simulink model "SWC_HALOUT_type"  (R2021b)
settings: Solver=FixedStepDiscrete  StartTime=0.0  StopTime=10.0  FixedStep=0.001  RelTol=1e-3
values from neighbouring files (symbols this model uses):
  DIDLen_APPPedalZP = uint16(3)    [vcu_local_hdr.m]
  DIDLen_APSFunConfig = uint16(16)    [vcu_local_hdr.m]
  DIDLen_AutoLock = uint16(1)    [vcu_local_hdr.m]
  DIDLen_AutoWipHSpdEN = uint16(1)    [vcu_local_hdr.m]
  DIDLen_DKCKey = uint16(8)    [vcu_local_hdr.m]
  DIDLen_DRLDis = uint16(1)    [vcu_local_hdr.m]
  DIDLen_DynoMode = uint16(1)    [vcu_local_hdr.m]
  DIDLen_FMHTimer = uint16(1)    [vcu_local_hdr.m]
  DIDLen_LFLowPresThre = uint16(1)    [vcu_local_hdr.m]
  DIDLen_LFSensorID = uint16(4)    [vcu_local_hdr.m]
  DIDLen_LRLowPresThre = uint16(1)    [vcu_local_hdr.m]
  DIDLen_LRSensorID = uint16(4)    [vcu_local_hdr.m]
  DIDLen_NVMPedalZP = uint16(3)    [vcu_local_hdr.m]
  DIDLen_RFLowPresThre = uint16(1)    [vcu_local_hdr.m]
  DIDLen_RFSensorID = uint16(4)    [vcu_local_hdr.m]
  DIDLen_RRLowPresThre = uint16(1)    [vcu_local_hdr.m]
  DIDLen_RRSensorID = uint16(4)    [vcu_local_hdr.m]
  DIDLen_SensorMode = uint16(1)    [vcu_local_hdr.m]
  DIDLen_TireSize = uint16(16)    [vcu_local_hdr.m]
  DIDLen_TPMSLearnSta = uint16(1)    [vcu_local_hdr.m]
  DIDLen_TurnLampFLThreCurr = uint16(1)    [vcu_local_hdr.m]
  DIDLen_TurnLampFRThreCurr = uint16(1)    [vcu_local_hdr.m]
  DIDLen_TurnLampRLThreCurr = uint16(1)    [vcu_local_hdr.m]
  DIDLen_TurnLampRRThreCurr = uint16(1)    [vcu_local_hdr.m]
  DIDLen_USSConfig = uint16(16)    [vcu_local_hdr.m]
  DIDLen_WhlPres = uint16(4)    [vcu_local_hdr.m]
  DIDLen_WhlSensorBattSta = uint16(1)    [vcu_local_hdr.m]
  DIDLen_WhlTmp = uint16(4)    [vcu_local_hdr.m]
  DIDLen_WipRLSCmdCutFilter = uint16(1)    [vcu_local_hdr.m]
  DIDLen_WipRLSCmdHoldFilter = uint16(1)    [vcu_local_hdr.m]
  DIDLen_XWDMode = uint16(1)    [vcu_local_hdr.m]
  DIDNum_APPPedalZP = uint16(0x0206)    [vcu_local_hdr.m]
  DIDNum_APSFunConfig = uint16(0x0903)    [vcu_local_hdr.m]
  DIDNum_AutoLock = uint16(0x0306)    [vcu_local_hdr.m]
  DIDNum_AutoWipHSpdEN = uint16(0x0308)    [vcu_local_hdr.m]
  DIDNum_DKCKey = uint16(0x0202)    [vcu_local_hdr.m]
  DIDNum_DRLDis = uint16(0x0307)    [vcu_local_hdr.m]
  DIDNum_DynoMode = uint16(0x0203)    [vcu_local_hdr.m]
  DIDNum_FMHTimer = uint16(0x0305)    [vcu_local_hdr.m]
  DIDNum_LFLowPresThre = uint16(0x0B08)    [vcu_local_hdr.m]
  DIDNum_LFSensorID = uint16(0x0B01)    [vcu_local_hdr.m]
  DIDNum_LRLowPresThre = uint16(0x0B0A)    [vcu_local_hdr.m]
  DIDNum_LRSensorID = uint16(0x0B03)    [vcu_local_hdr.m]
  DIDNum_NVMPedalZP = uint16(0x0207)    [vcu_local_hdr.m]
  DIDNum_RFLowPresThre = uint16(0x0B09)    [vcu_local_hdr.m]
  DIDNum_RFSensorID = uint16(0x0B02)    [vcu_local_hdr.m]
  DIDNum_RRLowPresThre = uint16(0x0B0B)    [vcu_local_hdr.m]
  DIDNum_RRSensorID = uint16(0x0B04)    [vcu_local_hdr.m]
  DIDNum_SensorMode = uint16(0x0B0C)    [vcu_local_hdr.m]
  DIDNum_TireSize = uint16(0x0902)    [vcu_local_hdr.m]
  DIDNum_TPMSLearnSta = uint16(0x0B0D)    [vcu_local_hdr.m]
  DIDNum_TurnLampFLThreCurr = uint16(0x0303)    [vcu_local_hdr.m]
  DIDNum_TurnLampFRThreCurr = uint16(0x0301)    [vcu_local_hdr.m]
  DIDNum_TurnLampRLThreCurr = uint16(0x0304)    [vcu_local_hdr.m]
  DIDNum_TurnLampRRThreCurr = uint16(0x0302)    [vcu_local_hdr.m]
  DIDNum_USSConfig = uint16(0x0901)    [vcu_local_hdr.m]
  DIDNum_WhlPres = uint16(0x0B05)    [vcu_local_hdr.m]
  DIDNum_WhlSensorBattSta = uint16(0x0B07)    [vcu_local_hdr.m]
  DIDNum_WhlTmp = uint16(0x0B06)    [vcu_local_hdr.m]
  DIDNum_WipRLSCmdCutFilter = uint16(0x030A)    [vcu_local_hdr.m]
  DIDNum_WipRLSCmdHoldFilter = uint16(0x0309)    [vcu_local_hdr.m]
  DIDNum_XWDMode = uint16(0x0201)    [vcu_local_hdr.m]
  ENUM_TPMSLearnStatus_LEARNED = uint8(  1  )    [vcu_local_hdr.m]
  ENUM_TPMSLearnStatus_LEARNFAIL = uint8(  2  )    [vcu_local_hdr.m]
  ENUM_TPMSLearnStatus_NOTLEARN = uint8(  0  )    [vcu_local_hdr.m]
  FALSE = boolean( 0 )    [vcu_local_hdr.m]    (also in vcu_local_hdrTA2.m)
  TRUE = boolean( 1 )    [vcu_local_hdr.m]    (also in vcu_local_hdrTA2.m)
  ZERO_INT = uint8(0)    [vcu_local_hdr.m]    (also in vcu_local_hdrTA2.m)
undefined symbols (not defined in the file or in its folder): f32_ApsOutVehSpdSig, R_DIDWriteCDD_CSOP_DIDSet_APPPedalZP, R_DIDWriteCDD_CSOP_DIDSet_APSFunConfig, R_DIDWriteCDD_CSOP_DIDSet_AutoLock, R_DIDWriteCDD_CSOP_DIDSet_AutoWipHSpdEN, R_DIDWriteCDD_CSOP_DIDSet_DKCKey, R_DIDWriteCDD_CSOP_DIDSet_DRLDis, R_DIDWriteCDD_CSOP_DIDSet_DynoMode, R_DIDWriteCDD_CSOP_DIDSet_FMHTimer, R_DIDWriteCDD_CSOP_DIDSet_LFLowPresThre, R_DIDWriteCDD_CSOP_DIDSet_LFSensorID, R_DIDWriteCDD_CSOP_DIDSet_LRLowPresThre, R_DIDWriteCDD_CSOP_DIDSet_LRSensorID, R_DIDWriteCDD_CSOP_DIDSet_NVMPedalZP, R_DIDWriteCDD_CSOP_DIDSet_RFLowPresThre, R_DIDWriteCDD_CSOP_DIDSet_RFSensorID, R_DIDWriteCDD_CSOP_DIDSet_RRLowPresThre, R_DIDWriteCDD_CSOP_DIDSet_RRSensorID, R_DIDWriteCDD_CSOP_DIDSet_SensorMode, R_DIDWriteCDD_CSOP_DIDSet_TireSize, R_DIDWriteCDD_CSOP_DIDSet_TPMSLearnSta, R_DIDWriteCDD_CSOP_DIDSet_TurnLampFLThreCurr, R_DIDWriteCDD_CSOP_DIDSet_TurnLampFRThreCurr, R_DIDWriteCDD_CSOP_DIDSet_TurnLampRLThreCurr, R_DIDWriteCDD_CSOP_DIDSet_TurnLampRRThreCurr, R_DIDWriteCDD_CSOP_DIDSet_USSConfig, R_DIDWriteCDD_CSOP_DIDSet_WhlPres, R_DIDWriteCDD_CSOP_DIDSet_WhlSensorBattSta, R_DIDWriteCDD_CSOP_DIDSet_WhlTmp, R_DIDWriteCDD_CSOP_DIDSet_WipRLSCmdCutFilter, R_DIDWriteCDD_CSOP_DIDSet_WipRLSCmdHoldFilter, R_DIDWriteCDD_CSOP_DIDSet_XWDMode, R_FDCCDD_Inner_CSOP_FDC_AppCallSleep, R_HALINCDD_CSOP_PAS_Handler, R_HALINCDD_CSOP_UDS_Main, R_HALOUT_APS_CSOP_ApsOutput, R_HALOUTCDD_CSOP_AppNmStateReq, R_HALOUTCDD_CSOP_ResetPedalZeroPosDone, R_HALOUTCDD_CSOP_SetAcoreRebootCmdACK, R_HALOUTCDD_CSOP_SetHazardIND, R_HALOUTCDD_CSOP_SetSysPwrStat, R_HALOUTCDD_CSOP_SleepRequest, R_HALOUTCDD_CSOP_TPMSSensorIDRegSetResults, R_IOExpOUT_CDD_CSOP_IOExpSetVal, R_J1939_CAN1_FD1_CE100_0_CSOP_Write_CAN1_FD1_CE100_0, R_J1939_CAN1_FD1_CE100_1_CSOP_Write_CAN1_FD1_CE100_1, R_NVMWriteCDD_Inner_NVM_WriteOperation, R_UDSCDD_CSOP_DdmRestartOperationCycle, R_WDGCDD_CSOP_Call_WDG_AppEnd, u16_DIDLen_APPPedalZP, u16_DIDLen_APSFunConfig, u16_DIDLen_AutoLock, u16_DIDLen_AutoWipHSpdEN, u16_DIDLen_DKCKey, u16_DIDLen_DRLDis, u16_DIDLen_DynoMode, u16_DIDLen_FMHTimer, u16_DIDLen_LFLowPresThre, u16_DIDLen_LFSensorID, u16_DIDLen_LRLowPresThre ... (+95)
libraries: FVT_lib x142, simulink x107, hdlsllib x6, hcu_lib x5, halout x1
(part 2 of 8)

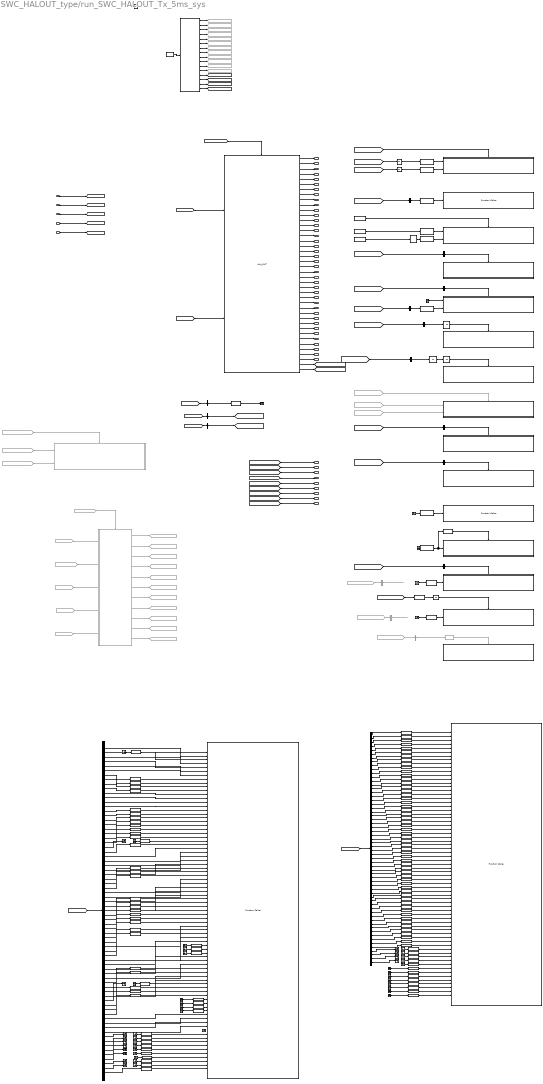
== system SWC_HALOUT_type/run_SWC_HALOUT_Tx_5ms_sys ==
  R_BSCP_outputs_BSCP_outputs_read : Inport
  R_BOUTP_outputs_BOUTP_outputs_read : Inport  Port=2
  R_BHAL_SYS_outputs_BHAL_SYS_outputs_read : Inport  Port=3
  R_BHAL_DID_outputs_BHAL_DID_outputs_read : Inport  Port=4
  R_NVMReadCDD_u8Array1024_NVMReadData_read : Inport  Port=5
  function : TriggerPort  TriggerType=function-call  VariantControl=(inherit)  SampleTimeType=periodic  SampleTime=-1
  Bus Selector1 : BusSelector  OutputSignals=VOUTP_triggerBAM_flg
  Bus Selector15 : BusSelector  OutputSignals=VHAL_AcoreReadyToSlp_flg
  Bus Selector2 : BusSelector  OutputSignals=VOUTP_triggerDT_flg
  Bus Selector3 : BusSelector  OutputSignals=VOUTP_BrkPedalPos_pct,VOUTP_ActAPSPosn_pct,VOUTP_LFRawWhlSpeed_kph,VOUTP_RFRawWhlSpeed_kph,VOUTP_LRRawWhlSpeed_kph,VOUTP_RRRawWhlSpeed_kph,VOUTP_LFRawWhlSpeedV_flg,VOUTP_RFRawWhlSpeedV_flg,VOUTP_LRRawWhlSpeedV_flg,VOUTP_RRRawWhlSpeedV_flg,VOUTP_LFWhlRotDir_enum,VOUTP_RFWhlRotDir_enum,VOUTP_LRWhlRotDir_enum,VOUTP_RRWhlRotDir_enum,VOUTP_LFPulseCountV_flg,VOUTP_RFPulseCountV_flg,VOUTP_LRPulseCountV_flg,VOUTP_RRPulseCountV_flg,VOUTP_LFPulseCount_enum,VOUTP_RFPulseCount_enum,VOUTP_LRPulseCount_enum,VOUTP_RRPulseCount_enum,VOUTP_VehSpeed_kph,VOUTP_APSCtrlAvail_flg,VOUTP_ShifterHandleCmd_enum,VOUTP_DriIntend_enum,VOUTP_EPSAOIControl_enum,VOUTP_SASAngle_Deg,VOUTP_SASSpeed_degps,VOUTP_SASSpeedValid_flg,VOUTP_SASCAL_flg,VOUTP_SASV_flg,VOUTP_GRADE_Deg,VOUTP_YawRate_degps,VOUTP_LatAccel_Gps,VOUTP_LongAccel_Gps,VOUTP_MCPressure_bar,VOUTP_YawRateV_flg,VOUTP_LatAccelV_flg,VOUTP_LongAccelV_flg,VOUTP_MCPressureV_bar,VOUTP_BrkSwSta_flg,VOUTP_BrkSwV_flg,VOUTP_ESCStandstill_flg,VOUTP_ESCAPSSta_enum,VOUTP_EPBExtReleaseAvail_flg,VOUTP_EPBExtApplyAvail_flg,VOUTP_EPBErrSta_enum,VOUTP_EPBSta_enum,VOUTP_AVMparkingcancel_enum,VOUTP_AVMparkingexcute_enum,VOUTP_AVMParkingmode_enum,VOUTP_AVMErrSTA_flg,VOUTP_IVIStatus_flg,VOUTP_CAASSw_enum,VOUTP_IVIScreen_enum,VOUTP_VehSpeedTimeOut_flg,VOUTP_ABSActive_flg,VOUTP_TCSActive_flg,VOUTP_DriverSeatBeltCmd_flg,VOUTP_RFPressIndi_enum,VOUTP_LFPressIndi_enum,VOUTP_RRPressIndi_enum,VOUTP_LRPressIndi_enum,VOUTP_FSOffSw_enum,VOUTP_FSOffSwTimeOut_flg,VOUTP_VehSpeed_kph,VOUTP_VehSpeed_kph,VOUTP_VehSpeed_kph,VOUTP_VehSpeed_kph,VOUTP_VehSpeed_kph,VOUTP_VehSpeed_kph,VOUTP_IVIUserTakeOverAPSSta_flg
  Bus Selector4 : BusSelector  OutputSignals=VOUTP_BrkPedalPosTimeOut_flg,VOUTP_LFRawWhlSpeedTimeOut_flg,VOUTP_RFRawWhlSpeedTimeOut_flg,VOUTP_LRRawWhlSpeedTimeOut_flg,VOUTP_RRRawWhlSpeedTimeOut_flg,VOUTP_LFRawWhlSpeedVTimeOut_flg,VOUTP_RFRawWhlSpeedVTimeOut_flg,VOUTP_LRRawWhlSpeedVTimeOut_flg,VOUTP_RRRawWhlSpeedVTimeOut_flg,VOUTP_LFWhlRotDirTimeOut_flg,VOUTP_RFWhlRotDirTimeOut_flg,VOUTP_LRWhlRotDirTimeOut_flg,VOUTP_RRWhlRotDirTimeOut_flg,VOUTP_LFPulseCountVTimeOut_flg,VOUTP_RFPulseCountVTimeOut_flg,VOUTP_LRPulseCountVTimeOut_flg,VOUTP_RRPulseCountVTimeOut_flg,VOUTP_LFPulseCountTimeOut_flg,VOUTP_RFPulseCountTimeOut_flg,VOUTP_LRPulseCountTimeOut_flg,VOUTP_RRPulseCountTimeOut_flg,VOUTP_ShifterHandleCmdTimeOut_flg,VOUTP_DriIntendTimeOut_flg,VOUTP_EPSAOIControlTimeOut_flg,VOUTP_SASAngleTimeOut_flg,VOUTP_SASSpeedTimeOut_flg,VOUTP_SASSpeedValidTimeOut_flg,VOUTP_SASCALTimeOut_flg,VOUTP_SASVTimeOut_flg,VOUTP_GRADETimeOut_flg,VOUTP_YawRateTimeOut_flg,VOUTP_LatAccelTimeOut_flg,VOUTP_LongAccelTimeOut_flg,VOUTP_MCPressureTimeOut_flg,VOUTP_YawRateVTimeOut_flg,VOUTP_LatAccelVTimeOut_flg,VOUTP_LongAccelVTimeOut_flg,VOUTP_MCPressureVTimeOut_flg,VOUTP_BrkSwStaTimeOut_flg,VOUTP_BrkSwVTimeOut_flg,VOUTP_ESCStandstillTimeOut_flg,VOUTP_ESCAPSStaTimeOut_flg,VOUTP_EPBExtReleaseAvailTimeOut_flg,VOUTP_EPBExtApplyAvailTimeOut_flg,VOUTP_EPBErrStaTimeOut_flg,VOUTP_EPBStaTimeOut_flg,VOUTP_AVMparkingcancelTimeOut_flg,VOUTP_AVMparkingexcuteTimeOut_flg,VOUTP_AVMParkingmodeTimeOut_flg,VOUTP_AVMErrSTATimeOut_flg,VOUTP_IVIStatusTimeOut_flg,VOUTP_CAASSwTimeOut_flg,VOUTP_IVIScreenTimeOut_flg,VOUTP_ABSActiveTimeOut_flg,VOUTP_TCSActiveTimeOut_flg,VOUTP_DriverSeatBeltCmdTimeOut_flg,VOUTP_RFPressIndi_enum,VOUTP_LFPressIndi_enum,VOUTP_RRPressIndi_enum,VOUTP_LRPressIndi_enum
  Bus Selector6 : BusSelector  Commented=on  OutputSignals=VHAL_TPMSSensorIDRegResults_raw8
  Bus Selector8 : BusSelector  Commented=on  OutputSignals=VOUTP_ResetPedalZeroPosStart_flg
  Bus Selector9 : BusSelector  Commented=on  OutputSignals=VHAL_DIDSetNVMPedalZP_raw8
  Constant2 : Constant  Value=TRUE
  Constant3 : Constant  Value=TRUE
  Constant4 : Constant  Value=TRUE
  Constant5 : Constant  Value=FALSE
  DIDSet_Subsystem : Subsystem  Commented=on
  DIDSet_Subsystem1 : From  Commented=on  GotoTag=BOUTP_DIDSetData_outputs
  DIDSet_Subsystem2 : From  Commented=on  GotoTag=BHAL_DID_outputs
  DIDSet_Subsystem3 : From  Commented=on  GotoTag=trig_SetDID
  Data Type Conversion{,1..2,4..5,7..13,17..19,21..107,109..125,128..130} (122 alike) : DataTypeConversion  OutDataTypeStr=uint8
  Data Type Conversion108 : DataTypeConversion  OutDataTypeStr=boolean
  Data Type Conversion126 : DataTypeConversion  OutDataTypeStr=boolean
  Data Type Conversion127 : DataTypeConversion  OutDataTypeStr=boolean
  Data Type Conversion{14..16,20} (4 alike) : DataTypeConversion  OutDataTypeStr=int16
  Data Type Conversion3 : DataTypeConversion  OutDataTypeStr=uint32
  Data Type Conversion6 : DataTypeConversion  OutDataTypeStr=single
  Detect Increase1 : simulink/Logic and Bit Operations/Detect Increase  Commented=on  vinit=0.0  OutDataTypeStr=boolean
  From104 : From  Commented=on  GotoTag=BHAL_SYS_outputs
  From118 : From  Commented=on  GotoTag=BHAL_SYS_outputs
  From121 : From  Commented=on  GotoTag=trig_OUTP_AFTER_40_1
  From122 : From  Commented=on  GotoTag=BOUTP_outputs
  From134 : From  Commented=on  GotoTag=BOUTP_DIDSetData_outputs
  From139 : From  Commented=on  GotoTag=BOUTP_outputs
  From144 : From  Commented=on  GotoTag=BOUTP_DIDSetData_outputs
  From18 : From  Commented=on  GotoTag=Header_Array
  From19 : From  Commented=on  GotoTag=DTC_Array
  From20 : From  Commented=on  GotoTag=DTC_Trigger
  From35 : From  Commented=on  GotoTag=u8Array1024_NvmReadArray
  From36 : From  Commented=on  GotoTag=BHAL_DID_outputs
  Goto10 : Goto  Commented=on  GotoTag=u8Array1024_NvmWriteArray
  Goto100 : Goto  Commented=on  GotoTag=trig_Read_NVM_00
  Goto102 : Goto  Commented=on  GotoTag=trig_ReadIMUOffset_00
  Goto105 : Goto  Commented=on  GotoTag=u8_ApsOutSetFrSensorOnCmd
  Goto106 : Goto  Commented=on  GotoTag=trig_GetNMID
  Goto107 : Goto  Commented=on  GotoTag=u8_ApsOutSetFrSensorSwTOCmd
  Goto108 : Goto  Commented=on  GotoTag=u8_ApsOutSetVehSpdTOCmd
  Goto109 : Goto  Commented=on  GotoTag=Header_Array
  Goto110 : Goto  Commented=on  GotoTag=u8_ApsOutSendChrgPlugSta
  Goto111 : Goto  Commented=on  GotoTag=f32_ApsOutVehSpdSig
  Goto113 : Goto  Commented=on  GotoTag=DTC_Array
  Goto119 : Goto  Commented=on  GotoTag=trig_HAL_DKC_10_3
  Goto121 : Goto  Commented=on  GotoTag=DTC_Trigger
  Goto122 : Goto  Commented=on  GotoTag=u8_ApsOutGearPosnSig
  Goto124 : Goto  Commented=on  GotoTag=BOUTP_DIDSetData_outputs
  Goto90 : Goto  Commented=on  GotoTag=trig_GetDID
  Goto91 : Goto  Commented=on  GotoTag=trig_WDG
  Goto92 : Goto  Commented=on  GotoTag=trig_HAL_DKC_10_2
  Goto93 : Goto  Commented=on  GotoTag=trig_HAL_CDD_10_1
  Goto96 : Goto  Commented=on  GotoTag=trig_OUTP_40
  Goto97 : Goto  Commented=on  GotoTag=trig_APP_30
  Goto98 : Goto  Commented=on  GotoTag=trig_INP_20
  Goto99 : Goto  Commented=on  GotoTag=trig_HAL_IN_10
  Ground{,1..18,20..21} (21 alike) : Ground
  Ground_{1,11..14,16..24,26,36..37} (17 alike) : Ground
  HALOUT_AFTER : Subsystem
  HAL_OUT : halout/HAL_OUT  SystemSampleTime=-1  VariantActivationTime=update diagram  Latency=0  AutoFrameSizeCalculation=off
  NOT : Logic  Operator=NOT  Inputs=1  AllPortsSameDT=off  OutDataTypeStr=boolean
  OUTP_AFTER : Subsystem  Commented=on
      settings: RTWSystemCode=Nonreusable function  RTWFcnNameOpts=Use subsystem name  RTWFileNameOpts=Use subsystem name
  R_DIDWriteCDD_CSOP_DIDSet_NVMPedalZP : Subsystem
  R_FDCCDD_Inner_CSOP_FDC_AppCallSleep : Subsystem
  R_HALOUTCDD_CSOP_AppNmStateReq : Subsystem
  R_HALOUTCDD_CSOP_ResetPedalZeroPosDone : Subsystem
  R_HALOUTCDD_CSOP_SetAcoreRebootCmdACK : Subsystem
  R_HALOUTCDD_CSOP_SetHazardIND : FunctionCaller  FunctionPrototype=R_HALOUTCDD_CSOP_SetHazardIND(u8_HazardIND)  InputArgumentSpecifications=uint8(1)
  R_HALOUTCDD_CSOP_SetSysPwrStat : FunctionCaller  FunctionPrototype=R_HALOUTCDD_CSOP_SetSysPwrStat(u8_SysPwrStat)  InputArgumentSpecifications=uint8(1)
  R_HALOUTCDD_CSOP_SleepRequest : Subsystem
  R_HALOUTCDD_CSOP_TPMSSensorIDRegSetResults : Subsystem
  R_HALOUT_APS_CSOP_ApsSetData : FunctionCaller  FunctionPrototype=R_HALOUT_APS_CSOP_ApsSetData(u8_SetPwrSta,f32_SetBrkPedalPos,f32_SetActAPSPosn,f32_SetLF_RawWhlSpeed,f32_SetRF_RawWhlSpeed,f32_SetLR_RawWhlSpeed,f32_SetRR_RawWhlSpeed,u8_SetLF_RawWhlSpeed_V,u8_SetRF_RawWhlSpeed_V,u8_SetLR_RawWhlSpeed_V,u8_SetRR_RawWhlSpeed_V,u8_SetLF_WhlRotDir,u8_SetRF_WhlRotDir,u8_SetLR_WhlRotDir,u8_SetRR_WhlRotDir,u8_SetLF_PulseCount_V,u8_SetRF_PulseCount_V,u8_SetLR_PulseCount_V,u8_SetRR_PulseCount_V,s16_SetLF_PulseCount,s16_SetRF_PulseCount,s16_SetLR_PulseCount,s16_SetRR_PulseCount,u8_SetAPS_Active,u8_SetAPS_CtrlAvail,u8_SetShifter_Handle_Cmd,u8_SetDriIntend,u8_SetEPS_AOI_Control,f32_SetSAS_Angle,f32_SetSAS_Speed,u8_SetSAS_Speed_Valid,u8_SetSAS_CAL,u8_SetSAS_OK,f32_SetGRADE,f32_SetYawRate,f32_SetLatAccel,f32_SetLongAccel,f32_SetMCPressure,u8_SetYawRate_V,u8_SetLatAccel_V,u8_SetLongAccel_V,u8_SetMCPressure_V,u8_SetBrkSw_Sta,u8_SetBrkSw_V,u8_SetESC_Standstill,u8_SetESC_APS_Sta,u8_SetEPBExtReleaseAvail,u8_SetEPBExtApplyAvail,u8_SetEPBErrSta,u8_SetEPBSta,u8_SetAllDoorSW,u8_SetHoodSW,u8_SetTailgate_SW,u8_SetAVM_parking_cancel,u8_SetAVM_parking_excute,u8_SetAVM_Parking_mode,u8_SetAVM_Err_STA,u8_SetIVI_Status,u8_SetCAAS_Sw,u8_SetIVI_Screen,u8_SetCAAS_CtrlAvail,u8_SetABS_Active,u8_SetTCS_Active,u8_SetDriverSeatBeltCmd,u8_SetDrDoorSW,u8_SetPsDoorSW,u8_SetRLDoorSW,u8_SetRRDoorSW,u8_SetRFPressIndi,u8_SetLFPressIndi,u8_SetRRPressIndi,u8_SetLRPressIndi,f32_SetsigAmbAirT,f32_SetVehActSpd,u8_SetCAAS_Active,u8_SetAPS_PwrReqAvail_sta,u8_SetDKC_PDkeyAreaRAPS_Sta,u8_SetDKC_ParkingMode_Cmd,u8_SetP_UID_LowPower,u8_SetDr_SeatSta,u8_SetVCU_RAPSErrLv2_flg,u8_SetVCU_RAPSErrLv3_flg,u8_SetIVI_UserTakeOver_APS_Sta)  InputArgumentSpecifications=uint8(1), single(1), single(1), single(1), single(1), single(1), single(1), uint8(1), uint8(1), uint8(1), uint8(1), uint8(1), uint8(1), uint8(1), uint8(1), uint8(1), uint8(1), uint8(1), uint8(1), int16(1), int16(1), int16(1), int16(1), uint8(1), uint8(1), uint8(1), uint8(1), uint8(1), single(1), single(1), uint8(1), uint8(1), uint8(1), single(1), single(1), single(1), single(1), single(1), uint8(1), uint8(1), uint8(1), uint8(1), uint8(1), uint8(1), uint8(1), uint8(1), uint8(1), uint8(1), uint8(1), uint8(1), uint8(1), uint8(1), uint8(1), uint8(1), uint8(1), uint8(1), uint8(1), uint8(1), uint8(1), uint8(1), uint8(1), uint8(1), uint8(1), uint8(1), uint8(1), uint8(1), uint8(1), uint8(1), uint8(1), uint8(1), uint8(1), uint8(1), single(1), single(1), uint8(1), uint8(1), uint8(1), uint8(1), uint8(1), uint8(1), uint8(1), uint8(1), uint8(1)
  R_HALOUT_APS_CSOP_ApsSetTimeout : FunctionCaller  FunctionPrototype=R_HALOUT_APS_CSOP_ApsSetTimeout(u8_SetBrkPedalPosTO,u8_SetLF_RawWhlSpeedTO,u8_SetRF_RawWhlSpeedTO,u8_SetLR_RawWhlSpeedTO,u8_SetRR_RawWhlSpeedTO,u8_SetLF_RawWhlSpeed_VTO,u8_SetRF_RawWhlSpeed_VTO,u8_SetLR_RawWhlSpeed_VTO,u8_SetRR_RawWhlSpeed_VTO,u8_SetLF_WhlRotDirTO,u8_SetRF_WhlRotDirTO,u8_SetLR_WhlRotDirTO,u8_SetRR_WhlRotDirTO,u8_SetLF_PulseCount_VTO,u8_SetRF_PulseCount_VTO,u8_SetLR_PulseCount_VTO,u8_SetRR_PulseCount_VTO,u8_SetLF_PulseCountTO,u8_SetRF_PulseCountTO,u8_SetLR_PulseCountTO,u8_SetRR_PulseCountTO,u8_SetShifter_Handle_CmdTO,u8_SetDriIntendTO,u8_SetEPS_AOI_ControlTO,u8_SetSAS_AngleTO,u8_SetSAS_SpeedTO,u8_SetSAS_Speed_ValidTO,u8_SetSAS_CALTO,u8_SetSAS_OKTO,u8_SetGRADETO,u8_SetYawRateTO,u8_SetLatAccelTO,u8_SetLongAccelTO,u8_SetMCPressureTO,u8_SetYawRate_VTO,u8_SetLatAccel_VTO,u8_SetLongAccel_VTO,u8_SetMCPressure_VTO,u8_SetBrkSw_StaTO,u8_SetBrkSw_VTO,u8_SetESC_StandstillTO,u8_SetESC_APS_StaTO,u8_SetEPBExtReleaseAvailTO,u8_SetEPBExtApplyAvailTO,u8_SetEPBErrStaTO,u8_SetEPBStaTO,u8_SetAVM_parking_cancelTO,u8_SetAVM_parking_excuteTO,u8_SetAVM_Parking_modeTO,u8_SetAVM_Err_STATO,u8_SetIVI_StatusTO,u8_SetCAAS_SwTO,u8_SetIVI_ScreenTO,u8_SetABS_ActiveTO,u8_SetTCS_ActiveTO,u8_SetDriverSeatBeltCmdTO,u8_SetRFPressIndiTO,u8_SetLFPressIndiTO,u8_SetRRPressIndiTO,u8_SetLRPressIndiTO,u8_SetsigAmbAirTTO,u8_SetAPS_PwrReqAvail_staTO,u8_SetDKC_PDkeyAreaRAPS_StaTO,u8_SetDKC_ParkingMode_CmdTO,u8_SetP_UID_LowPowerTO,u8_SetDr_SeatStaTO,u8_SetVCU_RAPSErrLv2_flgTO,u8_SetVCU_RAPSErrLv3_flgTO,u8_SetIVI_UserTakeOver_APS_StaTO)  InputArgumentSpecifications=uint8(1), uint8(1), uint8(1), uint8(1), uint8(1), uint8(1), uint8(1), uint8(1), uint8(1), uint8(1), uint8(1), uint8(1), uint8(1), uint8(1), uint8(1), uint8(1), uint8(1), uint8(1), uint8(1), uint8(1), uint8(1), uint8(1), uint8(1), uint8(1), uint8(1), uint8(1), uint8(1), uint8(1), uint8(1), uint8(1), uint8(1), uint8(1), uint8(1), uint8(1), uint8(1), uint8(1), uint8(1), uint8(1), uint8(1), uint8(1), uint8(1), uint8(1), uint8(1), uint8(1), uint8(1), uint8(1), uint8(1), uint8(1), uint8(1), uint8(1), uint8(1), uint8(1), uint8(1), uint8(1), uint8(1), uint8(1), uint8(1), uint8(1), uint8(1), uint8(1), uint8(1), uint8(1), uint8(1), uint8(1), uint8(1), uint8(1), uint8(1), uint8(1), uint8(1)
  R_IOExpOUT_CDD_CSOP_IOExpSetVal : Subsystem
  R_NVMWriteCDD_Inner_NVM_WriteOperation : Subsystem
  R_UDSCDD_CSOP_DdmRestartOperationCycle : Subsystem
  R_UDSCDD_CSOP_SetDTCStatus : Subsystem
  R_WDGCDD_CSOP_Call_WDG_AppEnd : Subsystem
  Terminator{,1..8,10..15} (15 alike) : Terminator
  Unit Delay{,1..5} (6 alike) : UnitDelay  SampleTime=-1  HasFrameUpgradeWarning=on
  bus_selector : BusSelector  OutputSignals=VOUTP_SysPowerMode_enum
  bus_selector10 : BusSelector  OutputSignals=VOUTP_AcoreRebootCmdACK_flg
  bus_selector14 : BusSelector  OutputSignals=VOUTP_TPMSSensorIDRegStart_flg
  bus_selector4 : BusSelector  OutputSignals=VOUTP_NvWriteReqRisingEdge_flg
  bus_selector5 : BusSelector  OutputSignals=VOUTP_FdcSlpTime_sec
  bus_selector6 : BusSelector  OutputSignals=VOUTP_FdcSlpReqRisingEdge_flg
  bus_selector7 : BusSelector  OutputSignals=VOUTP_FdcSlpReqRisingEdge_flg
  bus_selector8 : BusSelector  OutputSignals=VOUTP_FdcSlpReqRisingEdge_flg
  bus_selector9 : BusSelector  OutputSignals=VOUTP_EnterNewOperCyc_flg
  detect_change1 : simulink/Logic and Bit Operations/Detect Change  vinit=0  OutDataTypeStr=boolean
  hcu_main_sched : Stateflow chart  TreatAsAtomicUnit=on
  P_CAN1_FD1_CE100_2_CAN1_SG_FD1_CE100_2_write : Outport
  P_CAN2_FD2_CE100_0_CAN2_SG_FD2_CE100_0_write : Outport  Port=2
  P_CAN4_FD4_CE100_0_CAN4_SG_FD4_CE100_0_write : Outport  Port=3
  P_CAN4_FD4_CE100_1_CAN4_SG_FD4_CE100_1_write : Outport  Port=4
  P_CAN7_FD7_CE100_0_CAN7_SG_FD7_CE100_0_write : Outport  Port=5
  IRV_ms10_CAN1_SG_FD1_C10_0_write : Outport  Port=6  OutDataTypeStr=Bus: DT_CAN1_SG_FD1_C10_0  PortDimensions=1  BusOutputAsStruct=on
  IRV_ms10_CAN1_SG_FD1_C10_1_write : Outport  Port=7  OutDataTypeStr=Bus: DT_CAN1_SG_FD1_C10_1  PortDimensions=1  BusOutputAsStruct=on
  IRV_ms10_CAN2_SG_FD2_C10_0_write : Outport  Port=8  OutDataTypeStr=Bus: DT_CAN2_SG_FD2_C10_0  PortDimensions=1  BusOutputAsStruct=on
  IRV_ms10_CAN3_SG_FD3_C10_0_write : Outport  Port=9  OutDataTypeStr=Bus: DT_CAN3_SG_FD3_C10_0  PortDimensions=1  BusOutputAsStruct=on
  IRV_ms10_CAN3_SG_FD3_C10_1_write : Outport  Port=10  OutDataTypeStr=Bus: DT_CAN3_SG_FD3_C10_1  PortDimensions=1  BusOutputAsStruct=on
  IRV_ms10_CAN4_SG_FD4_C10_0_write : Outport  Port=11  OutDataTypeStr=Bus: DT_CAN4_SG_FD4_C10_0  PortDimensions=1  BusOutputAsStruct=on
  IRV_ms10_CAN7_SG_FD7_C10_0_write : Outport  Port=12  OutDataTypeStr=Bus: DT_CAN7_SG_FD7_C10_0  PortDimensions=1  BusOutputAsStruct=on
  IRV_ms100_CAN1_SG_FD1_C100_0_write : Outport  Port=13  OutDataTypeStr=Bus: DT_CAN1_SG_FD1_C100_0  PortDimensions=1  BusOutputAsStruct=on
  IRV_ms100_CAN1_SG_FD1_C100_1_write : Outport  Port=14  OutDataTypeStr=Bus: DT_CAN1_SG_FD1_C100_1  PortDimensions=1  BusOutputAsStruct=on
  IRV_ms100_CAN1_SG_FD1_C100_2_write : Outport  Port=15  OutDataTypeStr=Bus: DT_CAN1_SG_FD1_C100_2  PortDimensions=1  BusOutputAsStruct=on
  IRV_ms100_CAN1_SG_FD1_C100_3_write : Outport  Port=16  OutDataTypeStr=Bus: DT_CAN1_SG_FD1_C100_3  PortDimensions=1  BusOutputAsStruct=on
  IRV_ms100_CAN2_SG_GW2_C100_0_write : Outport  Port=17  OutDataTypeStr=Bus: DT_CAN2_SG_GW2_C100_0  PortDimensions=1  BusOutputAsStruct=on
  IRV_ms100_CAN3_SG_FD3_C100_0_write : Outport  Port=18  OutDataTypeStr=Bus: DT_CAN3_SG_FD3_C100_0  PortDimensions=1  BusOutputAsStruct=on
  IRV_ms100_CAN4_SG_FD4_C100_0_write : Outport  Port=19  OutDataTypeStr=Bus: DT_CAN4_SG_FD4_C100_0  PortDimensions=1  BusOutputAsStruct=on
  IRV_ms100_CAN5_SG_FD5_C100_0_write : Outport  Port=20  OutDataTypeStr=Bus: DT_CAN5_SG_FD5_C100_0  PortDimensions=1  BusOutputAsStruct=on
  IRV_ms100_CAN7_SG_FD7_C100_0_write : Outport  Port=21  OutDataTypeStr=Bus: DT_CAN7_SG_FD7_C100_0  PortDimensions=1  BusOutputAsStruct=on
  IRV_ms1000_CAN2_SG_FD2_C1000_0_write : Outport  Port=22  OutDataTypeStr=Bus: DT_CAN2_SG_FD2_C1000_0  PortDimensions=1  BusOutputAsStruct=on
  IRV_ms20_CAN1_SG_FD1_C20_0_write : Outport  Port=23  OutDataTypeStr=Bus: DT_CAN1_SG_FD1_C20_0  PortDimensions=1  BusOutputAsStruct=on
  IRV_ms200_CAN1_SG_FD1_C200_0_write : Outport  Port=24  OutDataTypeStr=Bus: DT_CAN1_SG_FD1_C200_0  PortDimensions=1  BusOutputAsStruct=on
  IRV_ms200_CAN2_SG_FD2_C200_0_write : Outport  Port=25  OutDataTypeStr=Bus: DT_CAN2_SG_FD2_C200_0  PortDimensions=1  BusOutputAsStruct=on
  IRV_ms200_CAN3_SG_FD3_C200_0_write : Outport  Port=26  OutDataTypeStr=Bus: DT_CAN3_SG_FD3_C200_0  PortDimensions=1  BusOutputAsStruct=on
  IRV_ms200_CAN3_SG_FD3_C200_1_write : Outport  Port=27  OutDataTypeStr=Bus: DT_CAN3_SG_FD3_C200_1  PortDimensions=1  BusOutputAsStruct=on
  IRV_ms200_CAN4_SG_FD4_C200_0_write : Outport  Port=28  OutDataTypeStr=Bus: DT_CAN4_SG_FD4_C200_0  PortDimensions=1  BusOutputAsStruct=on
  IRV_ms200_CAN5_SG_FD5_C200_0_write : Outport  Port=29  OutDataTypeStr=Bus: DT_CAN5_SG_FD5_C200_0  PortDimensions=1  BusOutputAsStruct=on
  IRV_ms200_CAN6_SG_FD6_C200_0_write : Outport  Port=30  OutDataTypeStr=Bus: DT_CAN6_SG_FD6_C200_0  PortDimensions=1  BusOutputAsStruct=on
  IRV_ms200_CAN7_SG_FD7_C200_0_write : Outport  Port=31  OutDataTypeStr=Bus: DT_CAN7_SG_FD7_C200_0  PortDimensions=1  BusOutputAsStruct=on
  IRV_ms250_CAN1_SG_FD1_C250_0_write : Outport  Port=32  OutDataTypeStr=Bus: DT_CAN1_SG_FD1_C250_0  PortDimensions=1  BusOutputAsStruct=on
  IRV_ms50_CAN1_SG_FD1_C50_0_write : Outport  Port=33  OutDataTypeStr=Bus: DT_CAN1_SG_FD1_C50_0  PortDimensions=1  BusOutputAsStruct=on
  IRV_ms50_CAN1_SG_FD1_C50_1_write : Outport  Port=34  OutDataTypeStr=Bus: DT_CAN1_SG_FD1_C50_1  PortDimensions=1  BusOutputAsStruct=on
  IRV_ms50_CAN2_SG_FD2_C50_0_write : Outport  Port=35  OutDataTypeStr=Bus: DT_CAN2_SG_FD2_C50_0  PortDimensions=1  BusOutputAsStruct=on
  IRV_ms50_CAN7_SG_FD7_C50_0_write : Outport  Port=36  OutDataTypeStr=Bus: DT_CAN7_SG_FD7_C50_0  PortDimensions=1  BusOutputAsStruct=on
  IRV_ms500_CAN2_SG_FD2_C500_0_write : Outport  Port=37  OutDataTypeStr=Bus: DT_CAN2_SG_FD2_C500_0  PortDimensions=1  BusOutputAsStruct=on
  IRV_ms5000_CAN1_SG_FD1_C5000_0_write : Outport  Port=38  OutDataTypeStr=Bus: DT_CAN1_SG_FD1_C5000_0  PortDimensions=1  BusOutputAsStruct=on
  IRV_ms5000_CAN1_SG_FD1_C5000_1_write : Outport  Port=39  OutDataTypeStr=Bus: DT_CAN1_SG_FD1_C5000_1  PortDimensions=1  BusOutputAsStruct=on
  IRV_ms80_CAN1_SG_FD1_C80_0_write : Outport  Port=40  OutDataTypeStr=Bus: DT_CAN1_SG_FD1_C80_0  PortDimensions=1  BusOutputAsStruct=on
  IRV_f32_ApsOutVehSpdSig_write : Outport  Port=41  OutDataTypeStr=single  PortDimensions=1
  IRV_u8Array1024_NvmWriteArray_write : Outport  Port=42  OutDataTypeStr=uint8  PortDimensions=1024
  IRV_u8_ApsOutGearPosnSig_write : Outport  Port=43  OutDataTypeStr=uint8  PortDimensions=1
  IRV_u8_ApsOutSendChrgPlugSta_write : Outport  Port=44  OutDataTypeStr=uint8  PortDimensions=1
  IRV_u8_ApsOutSetFrSensorOnCmd_write : Outport  Port=45  OutDataTypeStr=uint8  PortDimensions=1
  IRV_u8_ApsOutSetFrSensorSwTOCmd_write : Outport  Port=46  OutDataTypeStr=uint8  PortDimensions=1
  IRV_u8_ApsOutSetVehSpdTOCmd_write : Outport  Port=47  OutDataTypeStr=uint8  PortDimensions=1
  IRV_J1939_CAN1_SG_FD1_CE100_0_write : Outport  Port=48  OutDataTypeStr=Bus: DT_CAN1_SG_FD1_CE100_0  PortDimensions=1  BusOutputAsStruct=on
  IRV_J1939_CAN1_SG_FD1_CE100_1_write : Outport  Port=49  OutDataTypeStr=Bus: DT_CAN1_SG_FD1_CE100_1  PortDimensions=1  BusOutputAsStruct=on
  wires:
  [f32_ApsOutVehSpdSig] -> IRV_f32_ApsOutVehSpdSig_write/1
  [u8Array1024_NvmWriteArray] -> IRV_u8Array1024_NvmWriteArray_write/1
  [u8_ApsOutGearPosnSig] -> IRV_u8_ApsOutGearPosnSig_write/1
  [u8_ApsOutSendChrgPlugSta] -> IRV_u8_ApsOutSendChrgPlugSta_write/1
  [u8_ApsOutSetFrSensorOnCmd] -> IRV_u8_ApsOutSetFrSensorOnCmd_write/1
  [u8_ApsOutSetFrSensorSwTOCmd] -> IRV_u8_ApsOutSetFrSensorSwTOCmd_write/1
  [u8_ApsOutSetVehSpdTOCmd] -> IRV_u8_ApsOutSetVehSpdTOCmd_write/1
  [J1939_CAN1_SG_FD1_CE100_0] -> IRV_J1939_CAN1_SG_FD1_CE100_0_write/1
  [J1939_CAN1_SG_FD1_CE100_1] -> IRV_J1939_CAN1_SG_FD1_CE100_1_write/1
  Data Type Conversion/1 -> R_HALOUTCDD_CSOP_SetSysPwrStat/1
  bus_selector/1 -> Data Type Conversion/1  "<VOUTP_SysPowerMode_enum>"
  [BOUTP_outputs] -> bus_selector/1
  bus_selector4/1 -> R_NVMWriteCDD_Inner_NVM_WriteOperation/Enable  "<VOUTP_NvWriteReqRisingEdge_flg>"
  [BOUTP_outputs] -> bus_selector4/1
  Data Type Conversion3/1 -> R_HALOUTCDD_CSOP_SleepRequest/2(WakeUpTime)
  bus_selector5/1 -> Data Type Conversion3/1  "<VOUTP_FdcSlpTime_sec>"
  [BOUTP_outputs] -> bus_selector5/1
  bus_selector6/1 -> R_HALOUTCDD_CSOP_SleepRequest/Enable  "<VOUTP_FdcSlpReqRisingEdge_flg>"
  [BOUTP_outputs] -> bus_selector6/1
  Unit Delay/1 -> R_WDGCDD_CSOP_Call_WDG_AppEnd/Enable
  bus_selector7/1 -> Unit Delay/1  "<VOUTP_FdcSlpReqRisingEdge_flg>"
  [BOUTP_outputs] -> bus_selector7/1
  Unit Delay1/1 -> R_FDCCDD_Inner_CSOP_FDC_AppCallSleep/Enable
  Unit Delay2/1 -> Unit Delay1/1
  bus_selector8/1 -> Unit Delay2/1  "<VOUTP_FdcSlpReqRisingEdge_flg>"
  [BOUTP_outputs] -> bus_selector8/1
  From18/1 -> R_UDSCDD_CSOP_SetDTCStatus/1(Header_Array)
  From19/1 -> R_UDSCDD_CSOP_SetDTCStatus/2(DTC_Array)
  From20/1 -> R_UDSCDD_CSOP_SetDTCStatus/Enable
  bus_selector9/1 -> R_UDSCDD_CSOP_DdmRestartOperationCycle/Enable  "<VOUTP_EnterNewOperCyc_flg>"
  [BOUTP_outputs] -> bus_selector9/1
  bus_selector10/1 -> R_HALOUTCDD_CSOP_SetAcoreRebootCmdACK/Enable  "<VOUTP_AcoreRebootCmdACK_flg>"
  [BOUTP_outputs] -> bus_selector10/1
  Data Type Conversion4/1 -> R_HALOUTCDD_CSOP_SetHazardIND/1
  Data Type Conversion5/1 -> detect_change1/1, R_IOExpOUT_CDD_CSOP_IOExpSetVal/1(In1)
  detect_change1/1 -> R_IOExpOUT_CDD_CSOP_IOExpSetVal/Enable
  bus_selector14/1 -> R_HALOUTCDD_CSOP_TPMSSensorIDRegSetResults/Enable  "<VOUTP_TPMSSensorIDRegStart_flg>"
  [BOUTP_outputs] -> bus_selector14/1
  [trig_HAL_OUTAFTER_50_1] -> HALOUT_AFTER/Trigger
  DIDSet_Subsystem1/1 -> DIDSet_Subsystem/1(BOUTP_DIDSetData_outputs)
  DIDSet_Subsystem2/1 -> DIDSet_Subsystem/2(BHAL_DID_outputs)
  DIDSet_Subsystem3/1 -> DIDSet_Subsystem/Trigger
  hcu_main_sched/13(trig_OUTP_AFTER_40_1()) -> [trig_OUTP_AFTER_40_1]
  Constant5/1 -> hcu_main_sched/1(VHAL_FusionSchedReq_flg)
  hcu_main_sched/6(trig_HAL_IN_10()) -> Goto99/1
  hcu_main_sched/5(trig_GetDID()) -> Goto90/1
  hcu_main_sched/9(trig_HAL_DKC_10_3()) -> Goto119/1
  hcu_main_sched/2(trig_ReadIMUOffset_00()) -> Goto102/1
  hcu_main_sched/14(trig_SetDID()) -> [trig_SetDID]
  hcu_main_sched/7(trig_HAL_CDD_10_1()) -> Goto93/1
  hcu_main_sched/10(trig_INP_20()) -> Goto98/1
  hcu_main_sched/8(trig_HAL_DKC_10_2()) -> Goto92/1
  hcu_main_sched/4(trig_GetNMID()) -> Goto106/1
  hcu_main_sched/11(trig_APP_30()) -> Goto97/1
  hcu_main_sched/1(trig_Read_NVM_00()) -> Goto100/1
  hcu_main_sched/12(trig_OUTP_40()) -> Goto96/1
  hcu_main_sched/15(trig_HAL_OUT_50()) -> [trig_HAL_OUT_50]
  hcu_main_sched/16(trig_HAL_OUTAFTER_50_1()) -> [trig_HAL_OUTAFTER_50_1]
  hcu_main_sched/3(trig_WDG()) -> Goto91/1
  [BOUTP_outputs] -> HAL_OUT/1
  [trig_HAL_OUT_50] -> HAL_OUT/Trigger
  [BSCP_outputs] -> HAL_OUT/2
  Bus Selector3/73 -> Data Type Conversion117/1  "<VOUTP_IVIUserTakeOverAPSSta_flg>"
  Data Type Conversion35/1 -> R_HALOUT_APS_CSOP_ApsSetData/53
  Bus Selector3/54 -> Data Type Conversion37/1  "<VOUTP_IVIStatus_flg>"
  Bus Selector3/30 -> Data Type Conversion21/1  "<VOUTP_SASSpeedValid_flg>"
  Bus Selector3/20 -> Data Type Conversion14/1  "<VOUTP_RFPulseCount_enum>"
  Ground_11/1 -> Data Type Conversion118/1
  Bus Selector3/37 -> R_HALOUT_APS_CSOP_ApsSetData/38  "<VOUTP_MCPressure_bar>"
  Data Type Conversion16/1 -> R_HALOUT_APS_CSOP_ApsSetData/23
  Data Type Conversion120/1 -> R_HALOUT_APS_CSOP_ApsSetData/78
  Bus Selector3/31 -> Data Type Conversion22/1  "<VOUTP_SASCAL_flg>"
  Bus Selector3/15 -> Data Type Conversion10/1  "<VOUTP_LFPulseCountV_flg>"
  Bus Selector3/6 -> R_HALOUT_APS_CSOP_ApsSetData/7  "<VOUTP_RRRawWhlSpeed_kph>"
  Bus Selector3/45 -> R_HALOUT_APS_CSOP_ApsSetData/46  "<VOUTP_ESCAPSSta_enum>"
  Bus Selector3/69 -> Terminator12/1  "<VOUTP_VehSpeed_kph>"
  Data Type Conversion12/1 -> R_HALOUT_APS_CSOP_ApsSetData/18
  Bus Selector3/26 -> R_HALOUT_APS_CSOP_ApsSetData/27  "<VOUTP_DriIntend_enum>"
  Bus Selector3/22 -> Data Type Conversion16/1  "<VOUTP_RRPulseCount_enum>"
  Bus Selector3/14 -> R_HALOUT_APS_CSOP_ApsSetData/15  "<VOUTP_RRWhlRotDir_enum>"
  Bus Selector3/19 -> Data Type Conversion20/1  "<VOUTP_LFPulseCount_enum>"
  Data Type Conversion10/1 -> R_HALOUT_APS_CSOP_ApsSetData/16
  Data Type Conversion32/1 -> R_HALOUT_APS_CSOP_ApsSetData/48
  Bus Selector3/48 -> R_HALOUT_APS_CSOP_ApsSetData/49  "<VOUTP_EPBErrSta_enum>"
  Data Type Conversion118/1 -> R_HALOUT_APS_CSOP_ApsSetData/76
  Bus Selector3/55 -> R_HALOUT_APS_CSOP_ApsSetData/59  "<VOUTP_CAASSw_enum>"
  [BOUTP_outputs] -> Bus Selector3/1
  Bus Selector3/11 -> R_HALOUT_APS_CSOP_ApsSetData/12  "<VOUTP_LFWhlRotDir_enum>"
  Bus Selector3/43 -> Data Type Conversion29/1  "<VOUTP_BrkSwV_flg>"
  Ground/1 -> Data Type Conversion6/1
  Bus Selector3/70 -> Terminator11/1  "<VOUTP_VehSpeed_kph>"
  Bus Selector3/27 -> R_HALOUT_APS_CSOP_ApsSetData/28  "<VOUTP_EPSAOIControl_enum>"
  Data Type Conversion33/1 -> R_HALOUT_APS_CSOP_ApsSetData/51
  Data Type Conversion102/1 -> R_HALOUT_APS_CSOP_ApsSetData/64
  Bus Selector3/21 -> Data Type Conversion15/1  "<VOUTP_LRPulseCount_enum>"
  Ground_14/1 -> Data Type Conversion121/1
  Ground_13/1 -> Data Type Conversion120/1
  Bus Selector3/64 -> R_HALOUT_APS_CSOP_ApsSetData/72  "<VOUTP_LRPressIndi_enum>"
  Bus Selector3/1 -> R_HALOUT_APS_CSOP_ApsSetData/2  "<VOUTP_BrkPedalPos_pct>"
  Bus Selector3/17 -> Data Type Conversion12/1  "<VOUTP_LRPulseCountV_flg>"
  Data Type Conversion34/1 -> R_HALOUT_APS_CSOP_ApsSetData/52
  Bus Selector3/32 -> Data Type Conversion23/1  "<VOUTP_SASV_flg>"
  Bus Selector3/7 -> Data Type Conversion7/1  "<VOUTP_LFRawWhlSpeedV_flg>"
  Bus Selector3/50 -> R_HALOUT_APS_CSOP_ApsSetData/54  "<VOUTP_AVMparkingcancel_enum>"
  Bus Selector3/62 -> R_HALOUT_APS_CSOP_ApsSetData/70  "<VOUTP_LFPressIndi_enum>"
  Bus Selector3/72 -> Terminator14/1  "<VOUTP_VehSpeed_kph>"
  Data Type Conversion28/1 -> R_HALOUT_APS_CSOP_ApsSetData/43
  Data Type Conversion105/1 -> R_HALOUT_APS_CSOP_ApsSetData/61
  Bus Selector3/18 -> Data Type Conversion13/1  "<VOUTP_RRPulseCountV_flg>"
  Bus Selector3/39 -> Data Type Conversion25/1  "<VOUTP_LatAccelV_flg>"
  Ground_12/1 -> Data Type Conversion119/1
  Bus Selector3/4 -> R_HALOUT_APS_CSOP_ApsSetData/5  "<VOUTP_RFRawWhlSpeed_kph>"
  Bus Selector3/35 -> R_HALOUT_APS_CSOP_ApsSetData/36  "<VOUTP_LatAccel_Gps>"
  Data Type Conversion22/1 -> R_HALOUT_APS_CSOP_ApsSetData/32
  Bus Selector3/41 -> Data Type Conversion27/1  "<VOUTP_MCPressureV_bar>"
  Ground7/1 -> Data Type Conversion105/1
  Data Type Conversion11/1 -> R_HALOUT_APS_CSOP_ApsSetData/17
  Data Type Conversion30/1 -> R_HALOUT_APS_CSOP_ApsSetData/45
  Bus Selector3/67 -> Terminator15/1  "<VOUTP_VehSpeed_kph>"
  Bus Selector3/28 -> R_HALOUT_APS_CSOP_ApsSetData/29  "<VOUTP_SASAngle_Deg>"
  Data Type Conversion104/1 -> R_HALOUT_APS_CSOP_ApsSetData/62
  Bus Selector3/38 -> Data Type Conversion24/1  "<VOUTP_YawRateV_flg>"
  Bus Selector3/59 -> Data Type Conversion103/1  "<VOUTP_TCSActive_flg>"
  Data Type Conversion20/1 -> R_HALOUT_APS_CSOP_ApsSetData/20
  Data Type Conversion24/1 -> R_HALOUT_APS_CSOP_ApsSetData/39
  Bus Selector3/36 -> R_HALOUT_APS_CSOP_ApsSetData/37  "<VOUTP_LongAccel_Gps>"
  Data Type Conversion96/1 -> R_HALOUT_APS_CSOP_ApsSetData/75
  Bus Selector3/5 -> R_HALOUT_APS_CSOP_ApsSetData/6  "<VOUTP_LRRawWhlSpeed_kph>"
  Bus Selector3/29 -> R_HALOUT_APS_CSOP_ApsSetData/30  "<VOUTP_SASSpeed_degps>"
  Data Type Conversion27/1 -> R_HALOUT_APS_CSOP_ApsSetData/42
  Data Type Conversion36/1 -> R_HALOUT_APS_CSOP_ApsSetData/57
  Ground_16/1 -> Data Type Conversion122/1
  Bus Selector3/8 -> Data Type Conversion8/1  "<VOUTP_RFRawWhlSpeedV_flg>"
  Bus Selector3/10 -> Data Type Conversion19/1  "<VOUTP_RRRawWhlSpeedV_flg>"
  Bus Selector3/57 -> Terminator7/1  "<VOUTP_VehSpeedTimeOut_flg>"
  Bus Selector3/52 -> R_HALOUT_APS_CSOP_ApsSetData/56  "<VOUTP_AVMParkingmode_enum>"
  Data Type Conversion18/1 -> R_HALOUT_APS_CSOP_ApsSetData/25
  Bus Selector3/42 -> Data Type Conversion28/1  "<VOUTP_BrkSwSta_flg>"
  Bus Selector3/3 -> R_HALOUT_APS_CSOP_ApsSetData/4  "<VOUTP_LFRawWhlSpeed_kph>"
  Data Type Conversion8/1 -> R_HALOUT_APS_CSOP_ApsSetData/9
  Data Type Conversion26/1 -> R_HALOUT_APS_CSOP_ApsSetData/41
  Data Type Conversion29/1 -> R_HALOUT_APS_CSOP_ApsSetData/44
  Bus Selector3/51 -> R_HALOUT_APS_CSOP_ApsSetData/55  "<VOUTP_AVMparkingexcute_enum>"
  Data Type Conversion17/1 -> R_HALOUT_APS_CSOP_ApsSetData/24
  Data Type Conversion31/1 -> R_HALOUT_APS_CSOP_ApsSetData/47
  Bus Selector3/56 -> R_HALOUT_APS_CSOP_ApsSetData/60  "<VOUTP_IVIScreen_enum>"
  Bus Selector3/71 -> Terminator13/1  "<VOUTP_VehSpeed_kph>"
  Bus Selector3/23 -> Terminator8/1  "<VOUTP_VehSpeed_kph>"
  Bus Selector3/33 -> R_HALOUT_APS_CSOP_ApsSetData/34  "<VOUTP_GRADE_Deg>"
  Bus Selector3/44 -> Data Type Conversion30/1  "<VOUTP_ESCStandstill_flg>"
  Ground6/1 -> Data Type Conversion96/1
  Bus Selector3/25 -> R_HALOUT_APS_CSOP_ApsSetData/26  "<VOUTP_ShifterHandleCmd_enum>"
  Bus Selector3/24 -> Data Type Conversion18/1  "<VOUTP_APSCtrlAvail_flg>"
  Bus Selector3/47 -> Data Type Conversion32/1  "<VOUTP_EPBExtApplyAvail_flg>"
  Bus Selector3/2 -> R_HALOUT_APS_CSOP_ApsSetData/3  "<VOUTP_ActAPSPosn_pct>"
  Bus Selector3/34 -> R_HALOUT_APS_CSOP_ApsSetData/35  "<VOUTP_YawRate_degps>"
  Ground8/1 -> Data Type Conversion17/1
  Bus Selector3/65 -> Terminator1/1  "<VOUTP_FSOffSw_enum>"
  Ground11/1 -> Data Type Conversion98/1
  Data Type Conversion21/1 -> R_HALOUT_APS_CSOP_ApsSetData/31
  Data Type Conversion7/1 -> R_HALOUT_APS_CSOP_ApsSetData/8
  Ground15/1 -> Data Type Conversion33/1
  Data Type Conversion117/1 -> R_HALOUT_APS_CSOP_ApsSetData/83
  Data Type Conversion98/1 -> R_HALOUT_APS_CSOP_ApsSetData/65
  Ground_1/1 -> Data Type Conversion128/1
  Bus Selector3/12 -> R_HALOUT_APS_CSOP_ApsSetData/13  "<VOUTP_RFWhlRotDir_enum>"
  Data Type Conversion13/1 -> R_HALOUT_APS_CSOP_ApsSetData/19
  Bus Selector3/16 -> Data Type Conversion11/1  "<VOUTP_RFPulseCountV_flg>"
  Bus Selector3/40 -> Data Type Conversion26/1  "<VOUTP_LongAccelV_flg>"
  Data Type Conversion15/1 -> R_HALOUT_APS_CSOP_ApsSetData/22
  Data Type Conversion23/1 -> R_HALOUT_APS_CSOP_ApsSetData/33
  Bus Selector3/46 -> Data Type Conversion31/1  "<VOUTP_EPBExtReleaseAvail_flg>"
  Bus Selector3/63 -> R_HALOUT_APS_CSOP_ApsSetData/71  "<VOUTP_RRPressIndi_enum>"
  Data Type Conversion119/1 -> R_HALOUT_APS_CSOP_ApsSetData/77
  Ground_17/1 -> Data Type Conversion124/1
  Data Type Conversion6/1 -> R_HALOUT_APS_CSOP_ApsSetData/74
  Data Type Conversion9/1 -> R_HALOUT_APS_CSOP_ApsSetData/10
  Bus Selector3/60 -> Data Type Conversion102/1  "<VOUTP_DriverSeatBeltCmd_flg>"
  Data Type Conversion124/1 -> R_HALOUT_APS_CSOP_ApsSetData/82
  Data Type Conversion103/1 -> R_HALOUT_APS_CSOP_ApsSetData/63
  Data Type Conversion14/1 -> R_HALOUT_APS_CSOP_ApsSetData/21
  Ground14/1 -> Data Type Conversion101/1
  Data Type Conversion19/1 -> R_HALOUT_APS_CSOP_ApsSetData/11
  Data Type Conversion101/1 -> R_HALOUT_APS_CSOP_ApsSetData/68
  Bus Selector3/13 -> R_HALOUT_APS_CSOP_ApsSetData/14  "<VOUTP_LRWhlRotDir_enum>"
  Bus Selector3/53 -> Data Type Conversion36/1  "<VOUTP_AVMErrSTA_flg>"
  Ground13/1 -> Data Type Conversion100/1
  Data Type Conversion37/1 -> R_HALOUT_APS_CSOP_ApsSetData/58
  Ground12/1 -> Data Type Conversion99/1
  Ground9/1 -> Data Type Conversion129/1
  Data Type Conversion121/1 -> R_HALOUT_APS_CSOP_ApsSetData/79
  Bus Selector3/68 -> Terminator10/1  "<VOUTP_VehSpeed_kph>"
  Bus Selector3/66 -> Terminator6/1  "<VOUTP_FSOffSwTimeOut_flg>"
  Ground16/1 -> Data Type Conversion34/1
  Bus Selector3/58 -> Data Type Conversion104/1  "<VOUTP_ABSActive_flg>"
  Ground17/1 -> Data Type Conversion35/1
  Bus Selector3/61 -> R_HALOUT_APS_CSOP_ApsSetData/69  "<VOUTP_RFPressIndi_enum>"
  Data Type Conversion128/1 -> R_HALOUT_APS_CSOP_ApsSetData/80
  Data Type Conversion99/1 -> R_HALOUT_APS_CSOP_ApsSetData/66
  Data Type Conversion100/1 -> R_HALOUT_APS_CSOP_ApsSetData/67
  Data Type Conversion122/1 -> R_HALOUT_APS_CSOP_ApsSetData/81
  Data Type Conversion25/1 -> R_HALOUT_APS_CSOP_ApsSetData/40
  Data Type Conversion129/1 -> R_HALOUT_APS_CSOP_ApsSetData/1
  Bus Selector3/49 -> R_HALOUT_APS_CSOP_ApsSetData/50  "<VOUTP_EPBSta_enum>"
  Bus Selector3/9 -> Data Type Conversion9/1  "<VOUTP_LRRawWhlSpeedV_flg>"
  Bus Selector4/50 -> Data Type Conversion97/1  "<VOUTP_AVMErrSTATimeOut_flg>"
  Bus Selector4/25 -> Data Type Conversion59/1  "<VOUTP_SASAngleTimeOut_flg>"
  Bus Selector4/40 -> Data Type Conversion73/1  "<VOUTP_BrkSwVTimeOut_flg>"
  Bus Selector4/4 -> Data Type Conversion38/1  "<VOUTP_LRRawWhlSpeedTimeOut_flg>"
  Bus Selector4/15 -> Data Type Conversion48/1  "<VOUTP_RFPulseCountVTimeOut_flg>"
  Bus Selector4/51 -> Data Type Conversion87/1  "<VOUTP_IVIStatusTimeOut_flg>"
  Ground_20/1 -> Data Type Conversion112/1
  Data Type Conversion84/1 -> R_HALOUT_APS_CSOP_ApsSetTimeout/48
  Bus Selector4/44 -> Data Type Conversion78/1  "<VOUTP_EPBExtApplyAvailTimeOut_flg>"
  Data Type Conversion42/1 -> R_HALOUT_APS_CSOP_ApsSetTimeout/9
  Ground_22/1 -> Data Type Conversion110/1
  Bus Selector4/60 -> Terminator5/1  "<VOUTP_LRPressIndi_enum>"
  Data Type Conversion97/1 -> R_HALOUT_APS_CSOP_ApsSetTimeout/50
  Data Type Conversion48/1 -> R_HALOUT_APS_CSOP_ApsSetTimeout/15
  Data Type Conversion112/1 -> R_HALOUT_APS_CSOP_ApsSetTimeout/64
  Bus Selector4/22 -> Data Type Conversion57/1  "<VOUTP_ShifterHandleCmdTimeOut_flg>"
  Ground_24/1 -> Data Type Conversion115/1
  Bus Selector4/37 -> Data Type Conversion70/1  "<VOUTP_LongAccelVTimeOut_flg>"
  Data Type Conversion59/1 -> R_HALOUT_APS_CSOP_ApsSetTimeout/25
  Bus Selector4/54 -> Data Type Conversion82/1  "<VOUTP_ABSActiveTimeOut_flg>"
  Data Type Conversion109/1 -> R_HALOUT_APS_CSOP_ApsSetTimeout/62
  Data Type Conversion110/1 -> R_HALOUT_APS_CSOP_ApsSetTimeout/66
  Data Type Conversion116/1 -> R_HALOUT_APS_CSOP_ApsSetTimeout/67
  Data Type Conversion55/1 -> R_HALOUT_APS_CSOP_ApsSetTimeout/18
  Data Type Conversion69/1 -> R_HALOUT_APS_CSOP_ApsSetTimeout/36
  Data Type Conversion70/1 -> R_HALOUT_APS_CSOP_ApsSetTimeout/37
  Data Type Conversion85/1 -> R_HALOUT_APS_CSOP_ApsSetTimeout/55
  Data Type Conversion50/1 -> R_HALOUT_APS_CSOP_ApsSetTimeout/17
  Bus Selector4/3 -> Data Type Conversion51/1  "<VOUTP_RFRawWhlSpeedTimeOut_flg>"
  Bus Selector4/31 -> Data Type Conversion64/1  "<VOUTP_YawRateTimeOut_flg>"
  Data Type Conversion75/1 -> R_HALOUT_APS_CSOP_ApsSetTimeout/38
  Data Type Conversion65/1 -> R_HALOUT_APS_CSOP_ApsSetTimeout/28
  Data Type Conversion79/1 -> R_HALOUT_APS_CSOP_ApsSetTimeout/45
  Data Type Conversion82/1 -> R_HALOUT_APS_CSOP_ApsSetTimeout/54
  Bus Selector4/7 -> Data Type Conversion41/1  "<VOUTP_RFRawWhlSpeedVTimeOut_flg>"
  Bus Selector4/18 -> Data Type Conversion55/1  "<VOUTP_LFPulseCountTimeOut_flg>"
  Data Type Conversion86/1 -> R_HALOUT_APS_CSOP_ApsSetTimeout/49
  Ground_23/1 -> Data Type Conversion116/1
  Data Type Conversion57/1 -> R_HALOUT_APS_CSOP_ApsSetTimeout/22
  Bus Selector4/14 -> Data Type Conversion47/1  "<VOUTP_LFPulseCountVTimeOut_flg>"
  Bus Selector4/41 -> Data Type Conversion74/1  "<VOUTP_ESCStandstillTimeOut_flg>"
  Ground4/1 -> Data Type Conversion95/1
  Data Type Conversion123/1 -> R_HALOUT_APS_CSOP_ApsSetTimeout/2
  Bus Selector4/59 -> Terminator4/1  "<VOUTP_RRPressIndi_enum>"
  Data Type Conversion44/1 -> R_HALOUT_APS_CSOP_ApsSetTimeout/11
  Bus Selector4/17 -> Data Type Conversion50/1  "<VOUTP_RRPulseCountVTimeOut_flg>"
  Data Type Conversion54/1 -> R_HALOUT_APS_CSOP_ApsSetTimeout/21
  Bus Selector4/29 -> Data Type Conversion62/1  "<VOUTP_SASVTimeOut_flg>"
  Data Type Conversion114/1 -> R_HALOUT_APS_CSOP_ApsSetTimeout/69
  Bus Selector4/43 -> Data Type Conversion91/1  "<VOUTP_EPBExtReleaseAvailTimeOut_flg>"
  Data Type Conversion63/1 -> R_HALOUT_APS_CSOP_ApsSetTimeout/30
  Bus Selector4/23 -> Data Type Conversion71/1  "<VOUTP_DriIntendTimeOut_flg>"
  Bus Selector4/11 -> Data Type Conversion44/1  "<VOUTP_RFWhlRotDirTimeOut_flg>"
  Data Type Conversion73/1 -> R_HALOUT_APS_CSOP_ApsSetTimeout/40
  Data Type Conversion91/1 -> R_HALOUT_APS_CSOP_ApsSetTimeout/43
  Bus Selector4/33 -> Data Type Conversion76/1  "<VOUTP_LongAccelTimeOut_flg>"
  Data Type Conversion43/1 -> R_HALOUT_APS_CSOP_ApsSetTimeout/10
  Ground_21/1 -> Data Type Conversion111/1
  Bus Selector4/24 -> Data Type Conversion58/1  "<VOUTP_EPSAOIControlTimeOut_flg>"
  Bus Selector4/55 -> Data Type Conversion85/1  "<VOUTP_TCSActiveTimeOut_flg>"
  Data Type Conversion56/1 -> R_HALOUT_APS_CSOP_ApsSetTimeout/13
  Data Type Conversion95/1 -> R_HALOUT_APS_CSOP_ApsSetTimeout/58
  Data Type Conversion87/1 -> R_HALOUT_APS_CSOP_ApsSetTimeout/51
  Bus Selector4/46 -> Data Type Conversion80/1  "<VOUTP_EPBStaTimeOut_flg>"
  Bus Selector4/20 -> Data Type Conversion53/1  "<VOUTP_LRPulseCountTimeOut_flg>"
  Bus Selector4/10 -> Data Type Conversion43/1  "<VOUTP_LFWhlRotDirTimeOut_flg>"
  Data Type Conversion52/1 -> R_HALOUT_APS_CSOP_ApsSetTimeout/19
  Data Type Conversion46/1 -> R_HALOUT_APS_CSOP_ApsSetTimeout/12
  Data Type Conversion78/1 -> R_HALOUT_APS_CSOP_ApsSetTimeout/44
  Bus Selector4/47 -> Data Type Conversion83/1  "<VOUTP_AVMparkingcancelTimeOut_flg>"
  Bus Selector4/9 -> Data Type Conversion42/1  "<VOUTP_RRRawWhlSpeedVTimeOut_flg>"
  Bus Selector4/8 -> Data Type Conversion45/1  "<VOUTP_LRRawWhlSpeedVTimeOut_flg>"
  Bus Selector4/28 -> Data Type Conversion65/1  "<VOUTP_SASCALTimeOut_flg>"
  Data Type Conversion51/1 -> R_HALOUT_APS_CSOP_ApsSetTimeout/3
  Data Type Conversion58/1 -> R_HALOUT_APS_CSOP_ApsSetTimeout/24
  Bus Selector4/26 -> Data Type Conversion60/1  "<VOUTP_SASSpeedTimeOut_flg>"
  Data Type Conversion71/1 -> R_HALOUT_APS_CSOP_ApsSetTimeout/23
  Data Type Conversion77/1 -> R_HALOUT_APS_CSOP_ApsSetTimeout/42
  Bus Selector4/48 -> Data Type Conversion84/1  "<VOUTP_AVMparkingexcuteTimeOut_flg>"
  Data Type Conversion92/1 -> R_HALOUT_APS_CSOP_ApsSetTimeout/61
  Data Type Conversion115/1 -> R_HALOUT_APS_CSOP_ApsSetTimeout/68
  Bus Selector4/42 -> Data Type Conversion77/1  "<VOUTP_ESCAPSStaTimeOut_flg>"
  Bus Selector4/2 -> Data Type Conversion123/1  "<VOUTP_LFRawWhlSpeedTimeOut_flg>"
  Bus Selector4/57 -> Terminator2/1  "<VOUTP_RFPressIndi_enum>"
  Bus Selector4/30 -> Data Type Conversion63/1  "<VOUTP_GRADETimeOut_flg>"
  Data Type Conversion68/1 -> R_HALOUT_APS_CSOP_ApsSetTimeout/35
  Data Type Conversion111/1 -> R_HALOUT_APS_CSOP_ApsSetTimeout/65
  Data Type Conversion106/1 -> R_HALOUT_APS_CSOP_ApsSetTimeout/57
  Data Type Conversion80/1 -> R_HALOUT_APS_CSOP_ApsSetTimeout/46
  Data Type Conversion66/1 -> R_HALOUT_APS_CSOP_ApsSetTimeout/32
  Data Type Conversion39/1 -> R_HALOUT_APS_CSOP_ApsSetTimeout/5
  Data Type Conversion93/1 -> R_HALOUT_APS_CSOP_ApsSetTimeout/60
  Data Type Conversion72/1 -> R_HALOUT_APS_CSOP_ApsSetTimeout/39
  Bus Selector4/19 -> Data Type Conversion52/1  "<VOUTP_RFPulseCountTimeOut_flg>"
  Data Type Conversion89/1 -> R_HALOUT_APS_CSOP_ApsSetTimeout/53
  Ground2/1 -> Data Type Conversion93/1
  Data Type Conversion41/1 -> R_HALOUT_APS_CSOP_ApsSetTimeout/7
  Data Type Conversion90/1 -> R_HALOUT_APS_CSOP_ApsSetTimeout/56
  Data Type Conversion94/1 -> R_HALOUT_APS_CSOP_ApsSetTimeout/59
  Data Type Conversion81/1 -> R_HALOUT_APS_CSOP_ApsSetTimeout/1
  Data Type Conversion60/1 -> R_HALOUT_APS_CSOP_ApsSetTimeout/26
  Bus Selector4/49 -> Data Type Conversion86/1  "<VOUTP_AVMParkingmodeTimeOut_flg>"
  Bus Selector4/38 -> Data Type Conversion75/1  "<VOUTP_MCPressureVTimeOut_flg>"
  [BOUTP_outputs] -> Bus Selector4/1
  Data Type Conversion83/1 -> R_HALOUT_APS_CSOP_ApsSetTimeout/47
  Ground_18/1 -> Data Type Conversion109/1
  Bus Selector4/52 -> Data Type Conversion88/1  "<VOUTP_CAASSwTimeOut_flg>"
  Bus Selector4/35 -> Data Type Conversion68/1  "<VOUTP_YawRateVTimeOut_flg>"
  Ground_19/1 -> Data Type Conversion113/1
  Ground3/1 -> Data Type Conversion94/1
  Data Type Conversion113/1 -> R_HALOUT_APS_CSOP_ApsSetTimeout/63
  Data Type Conversion62/1 -> R_HALOUT_APS_CSOP_ApsSetTimeout/29
  Bus Selector4/16 -> Data Type Conversion49/1  "<VOUTP_LRPulseCountVTimeOut_flg>"
  Bus Selector4/12 -> Data Type Conversion46/1  "<VOUTP_LRWhlRotDirTimeOut_flg>"
  Data Type Conversion64/1 -> R_HALOUT_APS_CSOP_ApsSetTimeout/31
  Bus Selector4/32 -> Data Type Conversion66/1  "<VOUTP_LatAccelTimeOut_flg>"
  Bus Selector4/13 -> Data Type Conversion56/1  "<VOUTP_RRWhlRotDirTimeOut_flg>"
  Bus Selector4/27 -> Data Type Conversion61/1  "<VOUTP_SASSpeedValidTimeOut_flg>"
  Data Type Conversion38/1 -> R_HALOUT_APS_CSOP_ApsSetTimeout/4
  Bus Selector4/53 -> Data Type Conversion89/1  "<VOUTP_IVIScreenTimeOut_flg>"
  Bus Selector4/56 -> Data Type Conversion90/1  "<VOUTP_DriverSeatBeltCmdTimeOut_flg>"
  Bus Selector4/34 -> Data Type Conversion67/1  "<VOUTP_MCPressureTimeOut_flg>"
  Data Type Conversion76/1 -> R_HALOUT_APS_CSOP_ApsSetTimeout/33
  Data Type Conversion47/1 -> R_HALOUT_APS_CSOP_ApsSetTimeout/14
  Data Type Conversion53/1 -> R_HALOUT_APS_CSOP_ApsSetTimeout/20
  Data Type Conversion74/1 -> R_HALOUT_APS_CSOP_ApsSetTimeout/41
  Data Type Conversion49/1 -> R_HALOUT_APS_CSOP_ApsSetTimeout/16
  Bus Selector4/21 -> Data Type Conversion54/1  "<VOUTP_RRPulseCountTimeOut_flg>"
  Bus Selector4/45 -> Data Type Conversion79/1  "<VOUTP_EPBErrStaTimeOut_flg>"
  Data Type Conversion40/1 -> R_HALOUT_APS_CSOP_ApsSetTimeout/6
  Data Type Conversion67/1 -> R_HALOUT_APS_CSOP_ApsSetTimeout/34
  Bus Selector4/5 -> Data Type Conversion39/1  "<VOUTP_RRRawWhlSpeedTimeOut_flg>"
  Bus Selector4/36 -> Data Type Conversion69/1  "<VOUTP_LatAccelVTimeOut_flg>"
  Ground5/1 -> Data Type Conversion106/1
  Bus Selector4/58 -> Terminator3/1  "<VOUTP_LFPressIndi_enum>"
  Data Type Conversion88/1 -> R_HALOUT_APS_CSOP_ApsSetTimeout/52
  Bus Selector4/39 -> Data Type Conversion72/1  "<VOUTP_BrkSwStaTimeOut_flg>"
  Bus Selector4/6 -> Data Type Conversion40/1  "<VOUTP_LFRawWhlSpeedVTimeOut_flg>"
  Bus Selector4/1 -> Data Type Conversion81/1  "<VOUTP_BrkPedalPosTimeOut_flg>"
  Ground_26/1 -> Data Type Conversion114/1
  Data Type Conversion45/1 -> R_HALOUT_APS_CSOP_ApsSetTimeout/8
  Data Type Conversion61/1 -> R_HALOUT_APS_CSOP_ApsSetTimeout/27
  Ground1/1 -> Data Type Conversion92/1
  R_BSCP_outputs_BSCP_outputs_read/1 -> [BSCP_outputs]
  R_BHAL_DID_outputs_BHAL_DID_outputs_read/1 -> [BHAL_DID_outputs]
  R_BOUTP_outputs_BOUTP_outputs_read/1 -> [BOUTP_outputs]
  R_BHAL_SYS_outputs_BHAL_SYS_outputs_read/1 -> [BHAL_SYS_outputs]
  R_NVMReadCDD_u8Array1024_NVMReadData_read/1 -> [u8Array1024_NvmReadArray]
  [BHAL_SYS_outputs] -> Bus Selector15/1
  Bus Selector15/1 -> Data Type Conversion125/1  "<VHAL_AcoreReadyToSlp_flg>"
  Data Type Conversion125/1 -> Terminator/1
  Bus Selector2/1 -> [J1939_CAN1_FD1_CE100_0_Trigger]  "<VOUTP_triggerDT_flg>"
  [BOUTP_outputs] -> Bus Selector2/1
  Bus Selector1/1 -> [J1939_CAN1_FD1_CE100_1_Trigger]  "<VOUTP_triggerBAM_flg>"
  [BOUTP_outputs] -> Bus Selector1/1
  From118/1 -> OUTP_AFTER/3(BHAL_SYS_outputs)
  OUTP_AFTER/9(Header_Array) -> Goto109/1
  From122/1 -> OUTP_AFTER/1(BOUTP_outputs)
  OUTP_AFTER/10(DTC_Array) -> Goto113/1
  From104/1 -> OUTP_AFTER/2(BHAL_SYSTPMS_outputs)
  OUTP_AFTER/6(ApsOut_VehSpdSig) -> Goto111/1
  OUTP_AFTER/11(BOUTP_DIDSetData_outputs) -> Goto124/1
  OUTP_AFTER/1(ApsOut_GearPosnSig) -> Goto122/1
  OUTP_AFTER/8(DTC_Trigger) -> Goto121/1
  From121/1 -> OUTP_AFTER/Trigger
  OUTP_AFTER/5(ApsOut_SetVehSpdTOCmd) -> Goto108/1
  OUTP_AFTER/4(ApsOut_SetFrSensorSwTOCmd) -> Goto107/1
  OUTP_AFTER/2(ApsOut_SendChrgPlugStaSig) -> Goto110/1
  From36/1 -> OUTP_AFTER/5(BHAL_DIDGetData_raw)
  From35/1 -> OUTP_AFTER/4(VHAL_NvmReadArray_raw)
  OUTP_AFTER/7(HAL_NvmWriteData_raw) -> Goto10/1
  OUTP_AFTER/3(ApsOut_SetFrSensorOnCmd) -> Goto105/1
  [J1939_CAN1_FD1_CE100_1_Trigger] -> Unit Delay5/1
  [J1939_CAN1_FD1_CE100_0_Trigger] -> Unit Delay3/1
  Unit Delay5/1 -> Data Type Conversion127/1
  Unit Delay3/1 -> Data Type Conversion126/1
  Data Type Conversion126/1 -> HALOUT_AFTER/1(J1939_CAN1_FD1_CE100_0_Trigger)
  Data Type Conversion127/1 -> HALOUT_AFTER/2(J1939_CAN1_FD1_CE100_1_Trigger)
  Data Type Conversion2/1 -> R_HALOUTCDD_CSOP_AppNmStateReq/2(SleepReq)
  Constant4/1 -> NOT/1
  NOT/1 -> Data Type Conversion2/1
  Constant2/1 -> Data Type Conversion1/1
  Constant3/1 -> R_HALOUTCDD_CSOP_AppNmStateReq/Enable
  Data Type Conversion1/1 -> R_HALOUTCDD_CSOP_AppNmStateReq/1(WakeReq)
  Ground10/1 -> R_HALOUTCDD_CSOP_SleepRequest/1(SleepState)
  Ground18/1 -> Data Type Conversion4/1
  Ground_36/1 -> Data Type Conversion5/1
  Bus Selector9/1 -> ?  "<VHAL_DIDSetNVMPedalZP_raw8>"
  Data Type Conversion108/1 -> Unit Delay4/1
  [u8_ReadPedalZeroPosReq] -> Data Type Conversion108/1
  From139/1 -> Bus Selector8/1
  Bus Selector8/1 -> Detect Increase1/1  "<VOUTP_ResetPedalZeroPosStart_flg>"
  Ground21/1 -> Data Type Conversion130/1
  Unit Delay4/1 -> R_DIDWriteCDD_CSOP_DIDSet_NVMPedalZP/Enable
  Detect Increase1/1 -> R_HALOUTCDD_CSOP_ResetPedalZeroPosDone/Enable
  From144/1 -> Bus Selector9/1
  From134/1 -> Bus Selector6/1
  Bus Selector6/1 -> ?  "<VHAL_TPMSSensorIDRegResults_raw8>"
  Data Type Conversion107/1 -> R_HALOUTCDD_CSOP_TPMSSensorIDRegSetResults/1(In1)
  Ground20/1 -> Data Type Conversion107/1
  Data Type Conversion130/1 -> R_DIDWriteCDD_CSOP_DIDSet_NVMPedalZP/1(In3)
  HAL_OUT/1 -> P_CAN1_FD1_CE100_2_CAN1_SG_FD1_CE100_2_write/1
  HAL_OUT/2 -> P_CAN2_FD2_CE100_0_CAN2_SG_FD2_CE100_0_write/1
  HAL_OUT/3 -> P_CAN4_FD4_CE100_0_CAN4_SG_FD4_CE100_0_write/1
  HAL_OUT/4 -> P_CAN4_FD4_CE100_1_CAN4_SG_FD4_CE100_1_write/1
  HAL_OUT/5 -> P_CAN7_FD7_CE100_0_CAN7_SG_FD7_CE100_0_write/1
  HAL_OUT/6 -> IRV_ms10_CAN1_SG_FD1_C10_0_write/1
  HAL_OUT/7 -> IRV_ms10_CAN1_SG_FD1_C10_1_write/1
  HAL_OUT/8 -> IRV_ms10_CAN2_SG_FD2_C10_0_write/1
  HAL_OUT/9 -> IRV_ms10_CAN3_SG_FD3_C10_0_write/1
  HAL_OUT/10 -> IRV_ms10_CAN3_SG_FD3_C10_1_write/1
  HAL_OUT/11 -> IRV_ms10_CAN4_SG_FD4_C10_0_write/1
  HAL_OUT/12 -> IRV_ms10_CAN7_SG_FD7_C10_0_write/1
  HAL_OUT/13 -> IRV_ms100_CAN1_SG_FD1_C100_0_write/1
  HAL_OUT/14 -> IRV_ms100_CAN1_SG_FD1_C100_1_write/1
  HAL_OUT/15 -> IRV_ms100_CAN1_SG_FD1_C100_2_write/1
  HAL_OUT/16 -> IRV_ms100_CAN1_SG_FD1_C100_3_write/1
  HAL_OUT/17 -> IRV_ms100_CAN2_SG_GW2_C100_0_write/1
  HAL_OUT/18 -> IRV_ms100_CAN3_SG_FD3_C100_0_write/1
  HAL_OUT/19 -> IRV_ms100_CAN4_SG_FD4_C100_0_write/1
  HAL_OUT/20 -> IRV_ms100_CAN5_SG_FD5_C100_0_write/1
  HAL_OUT/21 -> IRV_ms100_CAN7_SG_FD7_C100_0_write/1
  HAL_OUT/22 -> IRV_ms1000_CAN2_SG_FD2_C1000_0_write/1
  HAL_OUT/23 -> IRV_ms20_CAN1_SG_FD1_C20_0_write/1
  HAL_OUT/24 -> IRV_ms200_CAN1_SG_FD1_C200_0_write/1
  HAL_OUT/25 -> IRV_ms200_CAN2_SG_FD2_C200_0_write/1
  HAL_OUT/26 -> IRV_ms200_CAN3_SG_FD3_C200_0_write/1
  HAL_OUT/27 -> IRV_ms200_CAN3_SG_FD3_C200_1_write/1
  HAL_OUT/28 -> IRV_ms200_CAN4_SG_FD4_C200_0_write/1
  HAL_OUT/29 -> IRV_ms200_CAN5_SG_FD5_C200_0_write/1
  HAL_OUT/30 -> IRV_ms200_CAN6_SG_FD6_C200_0_write/1
  HAL_OUT/31 -> IRV_ms200_CAN7_SG_FD7_C200_0_write/1
  HAL_OUT/32 -> IRV_ms250_CAN1_SG_FD1_C250_0_write/1
  HAL_OUT/33 -> IRV_ms50_CAN1_SG_FD1_C50_0_write/1
  HAL_OUT/34 -> IRV_ms50_CAN1_SG_FD1_C50_1_write/1
  HAL_OUT/35 -> IRV_ms50_CAN2_SG_FD2_C50_0_write/1
  HAL_OUT/36 -> IRV_ms50_CAN7_SG_FD7_C50_0_write/1
  HAL_OUT/37 -> IRV_ms500_CAN2_SG_FD2_C500_0_write/1
  HAL_OUT/38 -> IRV_ms5000_CAN1_SG_FD1_C5000_0_write/1
  HAL_OUT/39 -> IRV_ms5000_CAN1_SG_FD1_C5000_1_write/1
  HAL_OUT/40 -> IRV_ms80_CAN1_SG_FD1_C80_0_write/1
  HAL_OUT/41 -> [J1939_CAN1_SG_FD1_CE100_0]
  HAL_OUT/42 -> [J1939_CAN1_SG_FD1_CE100_1]
